simulink model "mainsim"  (R2022b)
settings: Solver=ode23tb  StartTime=0.0  StopTime=30  FixedStep=1e-2  RelTol=1e-3
undefined symbols (not defined in the file): g_vect, m, mixer, mixer_inv, omega0, q0
settings Model: Creator=Pietro Bruschi  LastModifiedBy=Pietro Bruschi

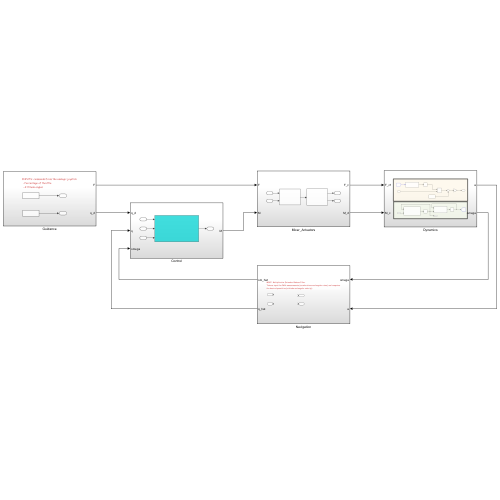
[thumbnail: Simulink's stored preview of the top-level diagram]
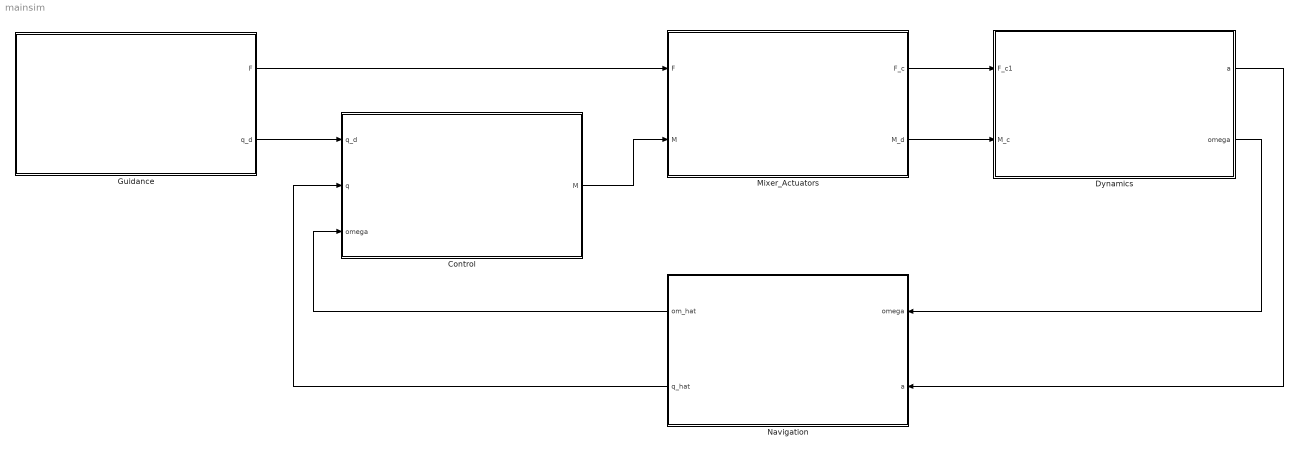
== system mainsim ==
  Control : Subsystem
  Dynamics : Subsystem
  Guidance : Subsystem
  Mixer_Actuators : Subsystem
  Navigation : Subsystem
      settings: PortSchema="{\"entries\":[{\"content\":{\"sides\":[{\"content\":{\"connectorIds\":[\"Out1\",\"Out2\"]},\"type\":\"ConnectorPlacement.EquallySpacedRectSide\",\"uuid\":\"6f66af9e-7d30-43a6-b817-d87f07ab7e88\"},{\"content\":{\"connectorIds\":[\"In1\",\"In2\"],\"side\":\"RIGHT\"},\"type\":\"ConnectorPlacement.EquallySpacedRectSide\",\"uuid\":\"d2c1230d-8f62-4a96-8f69-029e5818a673\"},{\"content\":{\"connectorIds\":[],\"side\":\"TOP\"},\"type\":\"ConnectorPlacement.EquallySpacedRectSide\",\"uuid\":\"6c3d714e-6440-4faf-82c6-25d40d07d2ee\"}]},\"type\":\"ConnectorPlacement.EquallySpacedConnector\",\"uuid\":\"c633ec09-2a70-434b-8cac-ea5e3c6390dc\"}],\"packageUris\":[\"http://schema.mathworks.com/mf0/Connector/R2020b\"],\"version\":\"1.0\"}"
  wires:
  Guidance/2(q_d) -> Control/1(q_d)
  Guidance/1(F) -> Mixer_Actuators/1(F)
  Control/1(M) -> Mixer_Actuators/2(M)
  Mixer_Actuators/1(F_c) -> Dynamics/1(F_c1)
  Mixer_Actuators/2(M_d) -> Dynamics/2(M_c)
  Dynamics/1(a) -> Navigation/2(a)
  Dynamics/2(omega) -> Navigation/1(omega)
  Navigation/1(om_hat) -> Control/3(omega)
  Navigation/2(q_hat) -> Control/2(q)

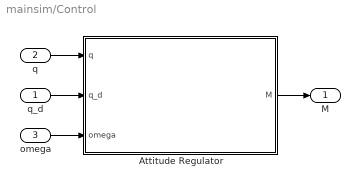
== system mainsim/Control ==
  q_d : Inport
  q : Inport  Port=2
  omega : Inport  Port=3
  Attitude Regulator : MATLAB Function  TreatAsAtomicUnit=on
  M : Outport
  wires:
  omega/1 -> Attitude Regulator/3(omega)
  q_d/1 -> Attitude Regulator/2(q_d)
  q/1 -> Attitude Regulator/1(q)
  Attitude Regulator/1(M) -> M/1

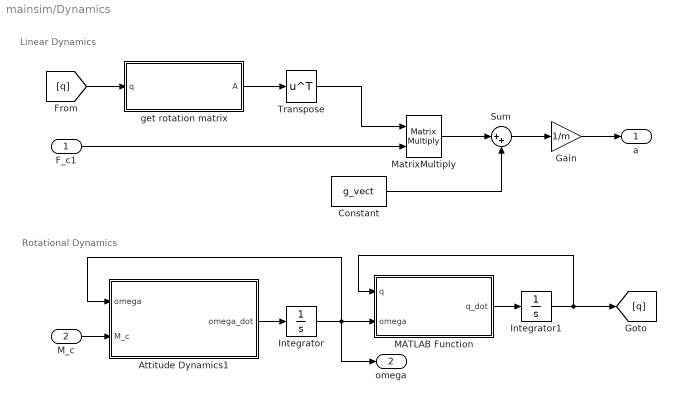
== system mainsim/Dynamics ==
  note: Rotational Dynamics
  note: Linear Dynamics
  F_c1 : Inport
  M_c : Inport  Port=2
  Attitude Dynamics1 : MATLAB Function  TreatAsAtomicUnit=on
  Constant : Constant  Value=g_vect
  Gain : Gain  Gain=1/m
  Integrator : Integrator  InitialCondition=omega0
  Integrator1 : Integrator  InitialCondition=q0
  MATLAB Function : MATLAB Function  TreatAsAtomicUnit=on
  MatrixMultiply : Product  Multiplication=Matrix(*)
  Sum : Sum  Inputs=|++
  Transpose : Math  Operator=transpose
  get rotation matrix : MATLAB Function  TreatAsAtomicUnit=on
  a : Outport
  omega : Outport  Port=2
  wires:
  M_c/1 -> Attitude Dynamics1/2(M_c)
  Attitude Dynamics1/1(omega_dot) -> Integrator/1
  Transpose/1 -> MatrixMultiply/1
  Sum/1 -> Gain/1
  F_c1/1 -> MatrixMultiply/2
  Constant/1 -> Sum/2
  MatrixMultiply/1 -> Sum/1
  get rotation matrix/1(A) -> Transpose/1
  [q] -> get rotation matrix/1(q)
  Gain/1 -> a/1
  MATLAB Function/1(q_dot) -> Integrator1/1
  Integrator1/1 -> [q], MATLAB Function/1(q)
  Integrator/1 -> MATLAB Function/2(omega), omega/1, Attitude Dynamics1/1(omega)

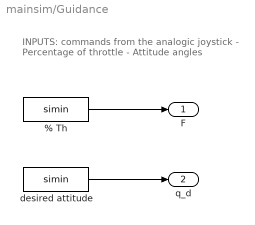
== system mainsim/Guidance ==
  note: INPUTS: commands from the analogic joystick
      | - Percentage of throttle
      | - Attitude angles
  % Th : FromWorkspace  VariableName=simin
  desired attitude : FromWorkspace  VariableName=simin
  F : Outport
  q_d : Outport  Port=2
  wires:
  % Th/1 -> F/1
  desired attitude/1 -> q_d/1

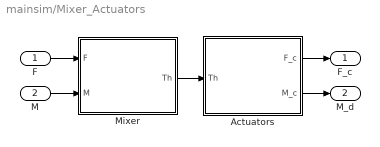
== system mainsim/Mixer_Actuators ==
  F : Inport
  M : Inport  Port=2
  Actuators : Subsystem
  Mixer : Subsystem
  F_c : Outport
  M_d : Outport  Port=2
  wires:
  F/1 -> Mixer/1(F)
  M/1 -> Mixer/2(M)
  Mixer/1(Th) -> Actuators/1(Th)
  Actuators/1(F_c) -> F_c/1
  Actuators/2(M_c) -> M_d/1

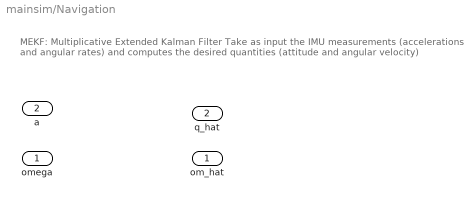
== system mainsim/Navigation ==
  note: MEKF: Multiplicative Extended Kalman Filter
      | Take as input the IMU measurements (accelerations and angular rates) and computes the desired quantities (attitude and angular velocity)
  omega : Inport
  a : Inport  Port=2
  om_hat : Outport
  q_hat : Outport  Port=2

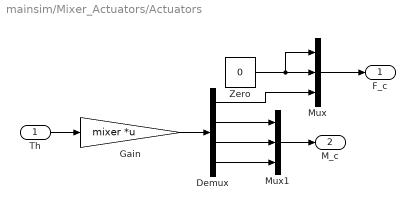
== system mainsim/Mixer_Actuators/Actuators ==
  Th : Inport
  Demux : Demux
  Gain : Gain  Gain=mixer  Multiplication=Matrix(K*u) (u vector)
  Mux : Mux  Inputs=3
  Mux1 : Mux  Inputs=3
  Zero : Constant  Value=0  OutDataTypeStr=Inherit: Inherit via back propagation
  F_c : Outport
  M_c : Outport  Port=2
  wires:
  Mux1/1 -> M_c/1
  Demux/2 -> Mux1/1
  Zero/1 -> Mux/1, Mux/2
  Mux/1 -> F_c/1
  Demux/4 -> Mux1/3
  Th/1 -> Gain/1
  Demux/1 -> Mux/3
  Gain/1 -> Demux/1
  Demux/3 -> Mux1/2

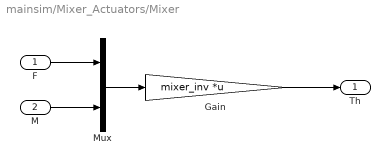
== system mainsim/Mixer_Actuators/Mixer ==
  F : Inport
  M : Inport  Port=2
  Gain : Gain  Gain=mixer_inv  Multiplication=Matrix(K*u) (u vector)
  Mux : Mux  Inputs=2
  Th : Outport
  wires:
  Mux/1 -> Gain/1
  F/1 -> Mux/1
  M/1 -> Mux/2
  Gain/1 -> Th/1

== matlab function mainsim/Dynamics/MATLAB Function ==
  data: q input; q_dot output; omega input
function q_dot = fcn(q, omega)

q = q/norm(q);

Omega = [       0   omega(3) -omega(2) omega(1) ;
         -omega(3)        0   omega(1) omega(2) ;
          omega(2) -omega(1)        0  omega(3) ;
         -omega(1) -omega(2) -omega(3)       0  ];

q_dot = 1/2 * Omega * q;

% Q = ...
% 
% q_dot = 1/2 * Q * omega;

== matlab function mainsim/Dynamics/Attitude Dynamics1 ==
  data: omega input; omega_dot output; M_c input; Drone parameter
function omega_dot = fcn(omega, M_c, Drone)

J = Drone.J;
Jinv = Drone.Jinv;

omega_dot = Jinv * (-cross(omega,J*omega) + M_c);

== matlab function mainsim/Dynamics/get rotation matrix ==
  data: q input; A output
function A = fcn(q)

q = q/norm(q);

q_v = q(1:3);

q_cross = [     0 -q(3)  q(2) ;
             q(3)     0 -q(1) ;
            -q(2)  q(1)     0 ];

A = (q(4) - q_v'*q_v)*eye(3) + 2*q_v*q_v' - 2*q(4)*q_cross;

% A = quat2dcm(q);

== matlab function mainsim/Control/Attitude Regulator ==
  data: q input; M output; q_d input; omega input; Controllers parameter
function M = fcn(q, q_d, omega, Controllers)

Kp_roll = Controllers.Kp_roll;
Kp_pitch = Controllers.Kp_pitch;
Kp_yaw = Controllers.Kp_yaw;
Kd_roll = Controllers.Kd_roll;
Kd_pitch = Controllers.Kd_pitch;
Kd_yaw = Controllers.Kd_yaw;

q_conj = [-q_d(1:3); q_d(4)];

Q = [  q(4)  q(3) -q(2)  q(1) ;
      -q(3)  q(4)  q(1)  q(2) ;
       q(2) -q(1)  q(4)  q(3) ; 
      -q(1) -q(2) -q(3)  q(4) ];

q_e = Q * q_conj;
q_e = q_e / norm(q_e);

M_x = 2*Kp_roll*(q_e(1)*q_e(4)) + Kd_roll*omega(1);
M_y = 2*Kp_pitch*(q_e(2)*q_e(4)) + Kd_pitch*omega(2);
M_z = 2*Kp_yaw*(q_e(3)*q_e(4)) + Kd_yaw*omega(3);

M = -[M_x M_y M_z]';
